simulink model "foc_host_serial_logger"  (R2025b)
settings: Solver=VariableStepAuto  StartTime=0.0  StopTime=inf  RelTol=1e-3
PostLoadFcn:
  | foc_sensorless_am13x_data;
values from neighbouring files (symbols this model uses):
  PU_System = mcb.getPUSystemParameters(pmsm, inverter)    [foc_sensorless_am13x_data.m]
  Ts = T_pwm    (= 5e-05)    [foc_sensorless_am13x_data.m]
libraries: instrumentseriallib x3, simulink x2
settings Model: Creator=a1255762  LastModifiedBy=a0542960

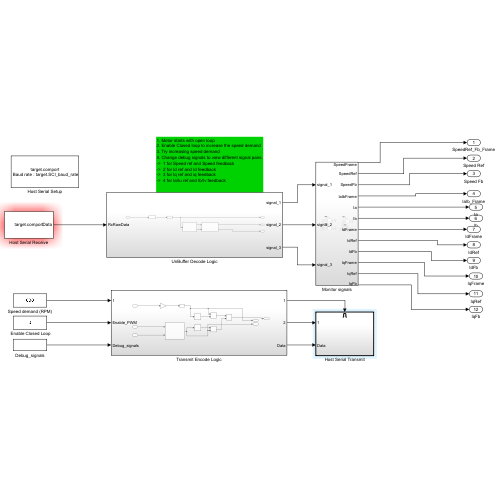
[thumbnail: Simulink's stored preview of the top-level diagram]
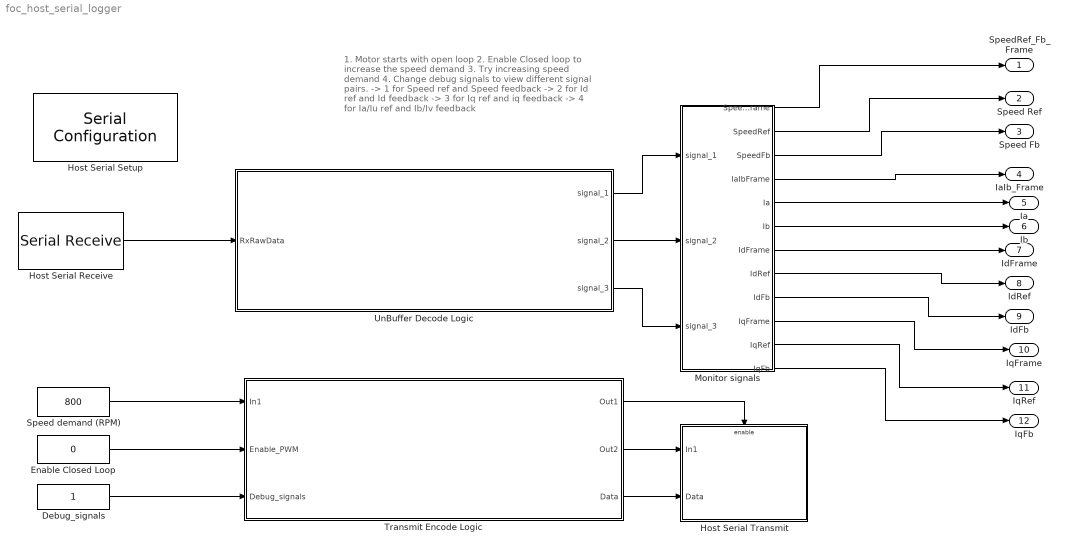
== system foc_host_serial_logger ==
  note: 1. Motor starts with open loop
      | 2. Enable Closed loop to increase the speed demand
      | 3. Try increasing speed demand
      | 4. Change debug signals to view different signal pairs.
      | ->  1 for Speed ref and Speed feedback
      | ->  2 for Id ref and Id feedback
      | ->  3 for Iq ref and iq feedback
      | ->  4 for Ia/Iu ref and Ib/Iv feedback
  " Enable Closed Loop" : Constant  Value=0  VectorParams1D=off  OutDataTypeStr=uint16  SampleTime=0.03
  Debug_signals : Constant  OutDataTypeStr=uint16  SampleTime=0.03
  Host Serial Receive : instrumentseriallib/Serial Receive  PortSel=target.comport  Port=target.comport  ComPort=target.comport  DataType=uint16  SaveDataType=uint8  ToggleHeader=off  Header='SS'  ToggleDataSize=on  DataSize=[600 2]  ToggleTerminator=on  Terminator=Custom terminator  CustomTerminator='EE'  InputFormat=Row major  EnableBlockingMode=on  ActionDataUnavailable=Output last received value  ActionWhenDataUnavailable=Output last received value  CustomValue=0  SampleTime=600 * Ts  SimulateUsing=Interpreted execution  BlockInModel=on  aMode=5  LibraryInUse=instrumentlib
  Host Serial Setup : instrumentseriallib/Serial Configuration  Priority=-99  PortSel=target.comport  Port=target.comport  ComPort=target.comport  BaudRate=target.SCI_baud_rate  DataBits=8  Parity=none  StopBits=1  ByteOrder=little-endian  FlowControl=none  Timeout=2  SimulateUsing=Interpreted execution  BlockInModel=on  aMode=5
      settings: LibrarySourceBlock=mcblib/Protection and Diagnostics/Host Serial Setup
  Host Serial Transmit : Subsystem  TreatAsAtomicUnit=on
  Monitor signals : Subsystem
  Speed demand (RPM) : Constant  Value=800  VectorParams1D=off  OutDataTypeStr=single  SampleTime=0.03
  Transmit Encode Logic : Subsystem
  UnBuffer Decode Logic : Subsystem
  SpeedRef_Fb_Frame : Outport
  Speed Ref : Outport  Port=2
  Speed Fb : Outport  Port=3
  IaIb_Frame : Outport  Port=4
  Ia : Outport  Port=5
  Ib : Outport  Port=6
  IdFrame : Outport  Port=7
  IdRef : Outport  Port=8
  IdFb : Outport  Port=9
  IqFrame : Outport  Port=10
  IqRef : Outport  Port=11
  IqFb : Outport  Port=12
  wires:
  Host Serial Receive/1 -> UnBuffer Decode Logic/1(RxRawData)
  Speed demand (RPM)/1 -> Transmit Encode Logic/1(In1)
  " Enable Closed Loop"/1 -> Transmit Encode Logic/2(Enable_PWM)
  Debug_signals/1 -> Transmit Encode Logic/3(Debug_signals)
  Transmit Encode Logic/1(Out1) -> Host Serial Transmit/Enable
  Transmit Encode Logic/2(Out2) -> Host Serial Transmit/1(In1)
  Transmit Encode Logic/3(Data) -> Host Serial Transmit/2(Data)
  UnBuffer Decode Logic/1(signal_1) -> Monitor signals/1(signal_1)
  UnBuffer Decode Logic/2(signal_2) -> Monitor signals/2(signal_2)
  UnBuffer Decode Logic/3(signal_3) -> Monitor signals/3(signal_3)
  Monitor signals/1(SpeedFrame) -> SpeedRef_Fb_Frame/1
  Monitor signals/2(SpeedRef) -> Speed Ref/1
  Monitor signals/3(SpeedFb) -> Speed Fb/1
  Monitor signals/4(IaIbFrame) -> IaIb_Frame/1
  Monitor signals/5(Ia) -> Ia/1
  Monitor signals/6(Ib) -> Ib/1
  Monitor signals/7(IdFrame) -> IdFrame/1
  Monitor signals/8(IdRef) -> IdRef/1
  Monitor signals/9(IdFb) -> IdFb/1
  Monitor signals/10(IqFrame) -> IqFrame/1
  Monitor signals/11(IqRef) -> IqRef/1
  Monitor signals/12(IqFb) -> IqFb/1

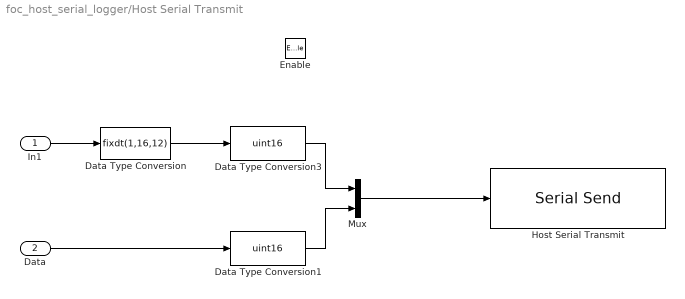
== system foc_host_serial_logger/Host Serial Transmit ==
  In1 : Inport
  Data : Inport  Port=2
  Enable : EnablePort
  Data Type Conversion : DataTypeConversion  OutDataTypeStr=fixdt(1,16,12)  RndMeth=Simplest  SaturateOnIntegerOverflow=off
  Data Type Conversion1 : DataTypeConversion  OutDataTypeStr=uint16  RndMeth=Simplest  SaturateOnIntegerOverflow=off
  Data Type Conversion3 : DataTypeConversion  OutDataTypeStr=uint16  ConvertRealWorld=Stored Integer (SI)  RndMeth=Simplest  SaturateOnIntegerOverflow=off
  Host Serial Transmit : instrumentseriallib/Serial Send  PortSel=target.comport  Port=target.comport  ComPort=target.comport  Header=[]  Terminator=<none>  CustomTerminator=[]  EnableBlockingMode=off  SimulateUsing=Interpreted execution  BlockInModel=on  aMode=5
  Mux : Mux  Inputs=2
  wires:
  Mux/1 -> Host Serial Transmit/1
  In1/1 -> Data Type Conversion/1
  Data Type Conversion/1 -> Data Type Conversion3/1
  Data Type Conversion3/1 -> Mux/1
  Data Type Conversion1/1 -> Mux/2
  Data/1 -> Data Type Conversion1/1

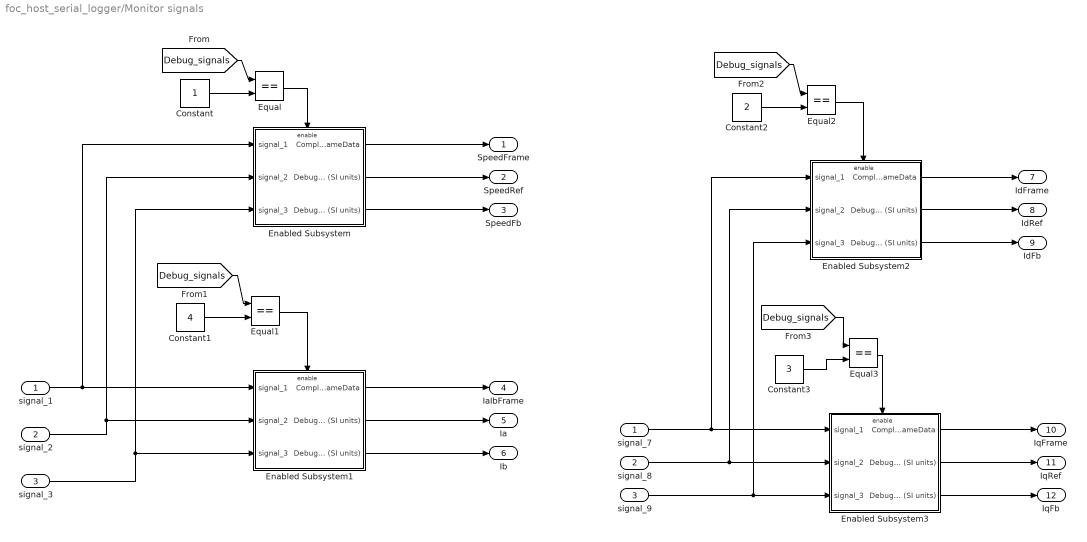
== system foc_host_serial_logger/Monitor signals ==
  signal_1 : Inport
  signal_2 : Inport  Port=2
  signal_3 : Inport  Port=3
  Constant : Constant
  Constant1 : Constant  Value=4
  Constant2 : Constant  Value=2
  Constant3 : Constant  Value=3
  Enabled Subsystem : Subsystem  TreatAsAtomicUnit=on
  Enabled Subsystem1 : Subsystem  TreatAsAtomicUnit=on
  Enabled Subsystem2 : Subsystem  TreatAsAtomicUnit=on
  Enabled Subsystem3 : Subsystem  TreatAsAtomicUnit=on
  Equal{,1..3} (4 alike) : RelationalOperator  Operator===  OutDataTypeStr=boolean  RndMeth=Simplest  InputSameDT=off
  signal_7 : InportShadow
  signal_8 : InportShadow  Port=2
  signal_9 : InportShadow  Port=3
  SpeedFrame : Outport
  SpeedRef : Outport  Port=2
  SpeedFb : Outport  Port=3
  IaIbFrame : Outport  Port=4
  Ia : Outport  Port=5
  Ib : Outport  Port=6
  IdFrame : Outport  Port=7
  IdRef : Outport  Port=8
  IdFb : Outport  Port=9
  IqFrame : Outport  Port=10
  IqRef : Outport  Port=11
  IqFb : Outport  Port=12
  wires:
  [Debug_signals] -> Equal1/1
  signal_2/1 -> Enabled Subsystem1/2(signal_2), Enabled Subsystem/2(signal_2)
  Enabled Subsystem1/2(Debug1 (SI units)) -> Ia/1
  signal_1/1 -> Enabled Subsystem1/1(signal_1), Enabled Subsystem/1(signal_1)
  Equal1/1 -> Enabled Subsystem1/Enable
  Constant/1 -> Equal/2
  [Debug_signals] -> Equal/1
  Constant1/1 -> Equal1/2
  signal_3/1 -> Enabled Subsystem1/3(signal_3), Enabled Subsystem/3(signal_3)
  Equal/1 -> Enabled Subsystem/Enable
  Enabled Subsystem1/1(CompleteFrameData) -> IaIbFrame/1
  Enabled Subsystem/2(Debug1 (SI units)) -> SpeedRef/1
  Enabled Subsystem1/3(Debug2 (SI units)) -> Ib/1
  Enabled Subsystem/1(CompleteFrameData) -> SpeedFrame/1
  Enabled Subsystem/3(Debug2 (SI units)) -> SpeedFb/1
  Enabled Subsystem2/3(Debug2 (SI units)) -> IdFb/1
  Enabled Subsystem2/1(CompleteFrameData) -> IdFrame/1
  Constant2/1 -> Equal2/2
  Equal2/1 -> Enabled Subsystem2/Enable
  Enabled Subsystem2/2(Debug1 (SI units)) -> IdRef/1
  [Debug_signals] -> Equal2/1
  [Debug_signals] -> Equal3/1
  Enabled Subsystem3/2(Debug1 (SI units)) -> IqRef/1
  Equal3/1 -> Enabled Subsystem3/Enable
  Constant3/1 -> Equal3/2
  Enabled Subsystem3/1(CompleteFrameData) -> IqFrame/1
  signal_7/1 -> Enabled Subsystem2/1(signal_1), Enabled Subsystem3/1(signal_1)
  signal_8/1 -> Enabled Subsystem2/2(signal_2), Enabled Subsystem3/2(signal_2)
  signal_9/1 -> Enabled Subsystem2/3(signal_3), Enabled Subsystem3/3(signal_3)
  Enabled Subsystem3/3(Debug2 (SI units)) -> IqFb/1

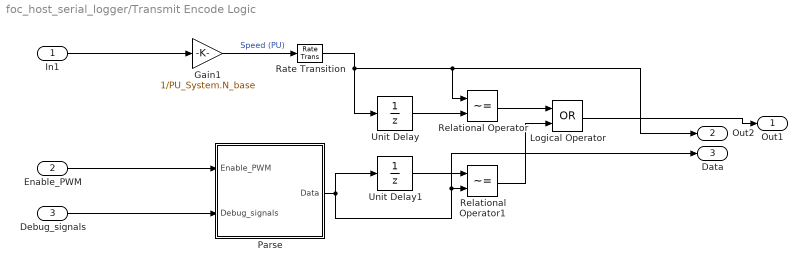
== system foc_host_serial_logger/Transmit Encode Logic ==
  In1 : Inport
  Enable_PWM : Inport  Port=2
  Debug_signals : Inport  Port=3
  Gain1 : Gain  Gain=1/PU_System.N_base  RndMeth=Simplest  OutDataTypeStr=Inherit: Same as input
  Logical Operator : Logic  Operator=OR  AllPortsSameDT=off  OutDataTypeStr=boolean
  Parse : Subsystem
  Rate Transition : RateTransition  OutPortSampleTime=0.03
  Relational Operator : RelationalOperator  Operator=~=  OutDataTypeStr=boolean  InputSameDT=off
  Relational Operator1 : RelationalOperator  Operator=~=  OutDataTypeStr=boolean  InputSameDT=off
  Unit Delay : UnitDelay  InitialCondition=0.5  SampleTime=-1  HasFrameUpgradeWarning=on
  Unit Delay1 : UnitDelay  SampleTime=-1  HasFrameUpgradeWarning=on
  Out1 : Outport
  Out2 : Outport  Port=2
  Data : Outport  Port=3
  wires:
  Logical Operator/1 -> Out1/1
  Parse/1(Data) -> Unit Delay1/1, Data/1, Relational Operator1/2
  Unit Delay/1 -> Relational Operator/2
  Unit Delay1/1 -> Relational Operator1/1
  Relational Operator1/1 -> Logical Operator/2
  Rate Transition/1 -> Unit Delay/1, Out2/1, Relational Operator/1
  Gain1/1 -> Rate Transition/1  "Speed (PU)"
  Relational Operator/1 -> Logical Operator/1
  In1/1 -> Gain1/1
  Debug_signals/1 -> Parse/2(Debug_signals)
  Enable_PWM/1 -> Parse/1(Enable_PWM)

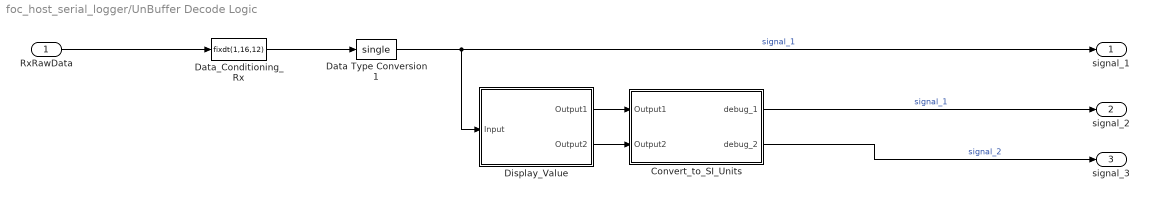
== system foc_host_serial_logger/UnBuffer Decode Logic ==
  RxRawData : Inport
  Convert_to_SI_Units : Subsystem
  Data Type Conversion1 : DataTypeConversion  OutDataTypeStr=single  RndMeth=Simplest  SaturateOnIntegerOverflow=off
  Data_Conditioning_Rx : DataTypeConversion  OutDataTypeStr=fixdt(1,16,12)  ConvertRealWorld=Stored Integer (SI)  RndMeth=Simplest  SaturateOnIntegerOverflow=off
  Display_Value : MATLAB Function  TreatAsAtomicUnit=on
  signal_1 : Outport
  signal_2 : Outport  Port=2
  signal_3 : Outport  Port=3
  wires:
  RxRawData/1 -> Data_Conditioning_Rx/1
  Data Type Conversion1/1 -> signal_1/1, Display_Value/1(Input)  "signal_1"
  Convert_to_SI_Units/1(debug_1) -> signal_2/1  "signal_1"
  Convert_to_SI_Units/2(debug_2) -> signal_3/1  "signal_2"
  Display_Value/2(Output2) -> Convert_to_SI_Units/2(Output2)
  Data_Conditioning_Rx/1 -> Data Type Conversion1/1
  Display_Value/1(Output1) -> Convert_to_SI_Units/1(Output1)

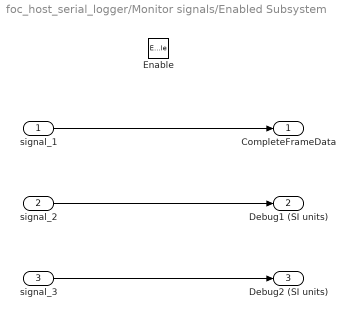
== system foc_host_serial_logger/Monitor signals/Enabled Subsystem ==
  signal_1 : Inport
  signal_2 : Inport  Port=2
  signal_3 : Inport  Port=3
  Enable : EnablePort
  CompleteFrameData : Outport  InitialOutput=0
  Debug1 (SI units) : Outport  Port=2  InitialOutput=0
  Debug2 (SI units) : Outport  Port=3  InitialOutput=0
  wires:
  signal_1/1 -> CompleteFrameData/1
  signal_2/1 -> Debug1 (SI units)/1
  signal_3/1 -> Debug2 (SI units)/1

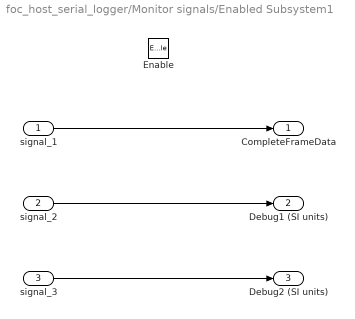
== system foc_host_serial_logger/Monitor signals/Enabled Subsystem1 ==
  signal_1 : Inport
  signal_2 : Inport  Port=2
  signal_3 : Inport  Port=3
  Enable : EnablePort
  CompleteFrameData : Outport  InitialOutput=0
  Debug1 (SI units) : Outport  Port=2  InitialOutput=0
  Debug2 (SI units) : Outport  Port=3  InitialOutput=0
  wires:
  signal_3/1 -> Debug2 (SI units)/1
  signal_2/1 -> Debug1 (SI units)/1
  signal_1/1 -> CompleteFrameData/1

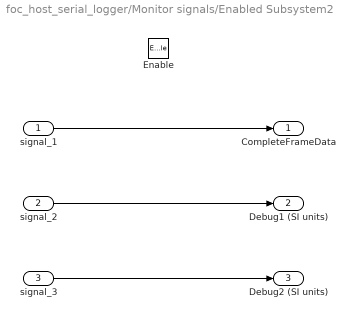
== system foc_host_serial_logger/Monitor signals/Enabled Subsystem2 ==
  signal_1 : Inport
  signal_2 : Inport  Port=2
  signal_3 : Inport  Port=3
  Enable : EnablePort
  CompleteFrameData : Outport  InitialOutput=0
  Debug1 (SI units) : Outport  Port=2  InitialOutput=0
  Debug2 (SI units) : Outport  Port=3  InitialOutput=0
  wires:
  signal_1/1 -> CompleteFrameData/1
  signal_2/1 -> Debug1 (SI units)/1
  signal_3/1 -> Debug2 (SI units)/1

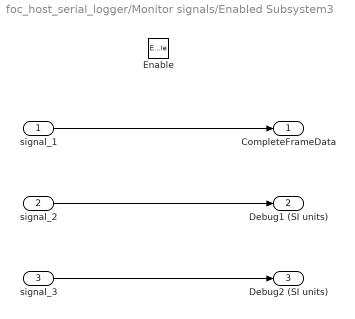
== system foc_host_serial_logger/Monitor signals/Enabled Subsystem3 ==
  signal_1 : Inport
  signal_2 : Inport  Port=2
  signal_3 : Inport  Port=3
  Enable : EnablePort
  CompleteFrameData : Outport  InitialOutput=0
  Debug1 (SI units) : Outport  Port=2  InitialOutput=0
  Debug2 (SI units) : Outport  Port=3  InitialOutput=0
  wires:
  signal_3/1 -> Debug2 (SI units)/1
  signal_2/1 -> Debug1 (SI units)/1
  signal_1/1 -> CompleteFrameData/1

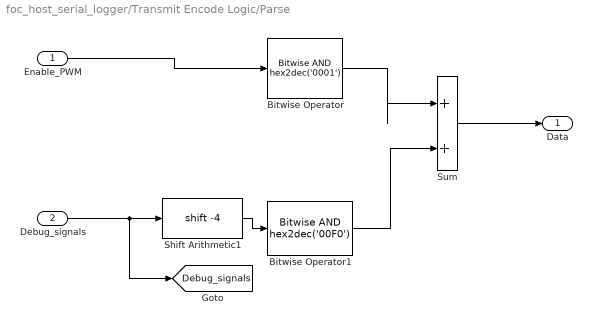
== system foc_host_serial_logger/Transmit Encode Logic/Parse ==
  Enable_PWM : Inport
  Debug_signals : Inport  Port=2
  Bitwise Operator : simulink/Logic and Bit Operations/Bitwise Operator  logicop=AND  UseBitMask=on  BitMask=hex2dec('0001')  BitMaskRealWorld=Stored Integer
  Bitwise Operator1 : simulink/Logic and Bit Operations/Bitwise Operator  logicop=AND  UseBitMask=on  BitMask=hex2dec('00F0')  BitMaskRealWorld=Stored Integer
  Shift Arithmetic1 : ArithShift  BitShiftNumber=-4
  Sum : Sum  Inputs=|++
  Data : Outport
  tag scope: Debug_signals=global
  wires:
  Bitwise Operator/1 -> Sum/1
  Debug_signals/1 -> [Debug_signals], Shift Arithmetic1/1
  Sum/1 -> Data/1
  Shift Arithmetic1/1 -> Bitwise Operator1/1
  Bitwise Operator1/1 -> Sum/2
  Enable_PWM/1 -> Bitwise Operator/1

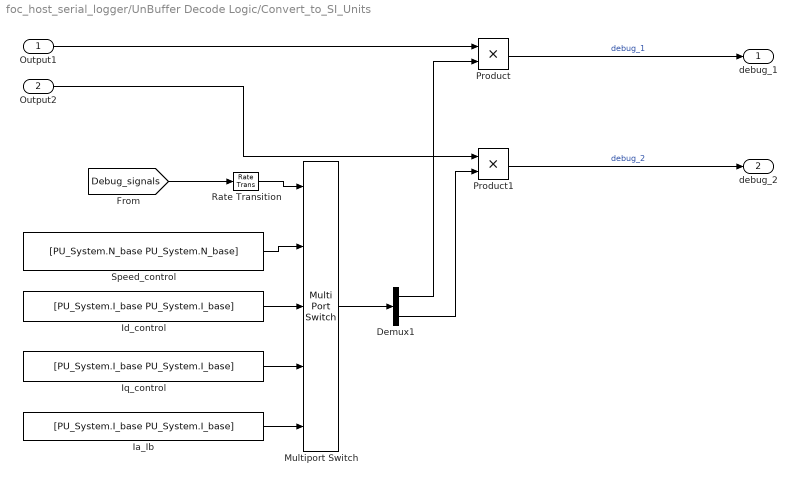
== system foc_host_serial_logger/UnBuffer Decode Logic/Convert_to_SI_Units ==
  Output1 : Inport
  Output2 : Inport  Port=2
  Demux1 : Demux  Outputs=2
  Ia_Ib : Constant  Value=[PU_System.I_base PU_System.I_base]  OutDataTypeStr=single  SampleTime=-1
  Id_control : Constant  Value=[PU_System.I_base PU_System.I_base]  OutDataTypeStr=single  SampleTime=-1
  Iq_control : Constant  Value=[PU_System.I_base PU_System.I_base]  OutDataTypeStr=single  SampleTime=-1
  Multiport Switch : MultiPortSwitch  Inputs=4  DiagnosticForDefault=Warning  OutDataTypeStr=single  RndMeth=Simplest  SaturateOnIntegerOverflow=off  InputSameDT=off
  Product : Product
  Product1 : Product
  Rate Transition : RateTransition  Deterministic=off
  Speed_control : Constant  Value=[PU_System.N_base PU_System.N_base]  OutDataTypeStr=single  SampleTime=-1
  debug_1 : Outport
  debug_2 : Outport  Port=2
  wires:
  Product/1 -> debug_1/1  "debug_1"
  Product1/1 -> debug_2/1  "debug_2"
  Id_control/1 -> Multiport Switch/3
  Speed_control/1 -> Multiport Switch/2
  Multiport Switch/1 -> Demux1/1
  Iq_control/1 -> Multiport Switch/4
  Demux1/2 -> Product1/2
  Demux1/1 -> Product/2
  Ia_Ib/1 -> Multiport Switch/5
  Output1/1 -> Product/1
  Output2/1 -> Product1/1
  Rate Transition/1 -> Multiport Switch/1
  [Debug_signals] -> Rate Transition/1

== matlab function foc_host_serial_logger/UnBuffer Decode Logic/Display_Value ==
  data: Output1 output; Output2 output; Input input
function [ Output1, Output2] = unBuf(Input)
%% ************************************************************************
% Unbuffer function
% Outputs first received serial data from buffer for both signals

% Copyright 2020 The MathWorks, Inc.

selSignal= Input(:, 1);
Output1 = selSignal(1,1);
selSignal = Input(:, 2);
Output2 = selSignal(1,1);
end
